simulink model "d2017_10_18_Pendulum"  (R2017b)
settings: Solver=VariableStepAuto  StartTime=0.0  StopTime=30.0  MaxStep=0.01  RelTol=1e-3
settings Model: Creator=ppolcz  LastModifiedBy=ppolcz

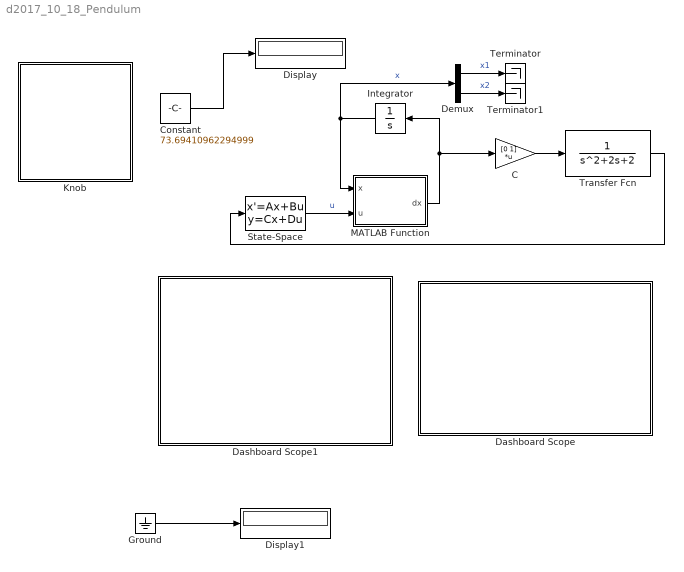
== system d2017_10_18_Pendulum ==
  C : Gain  Gain=[0 1]  Multiplication=Matrix(K*u)
  Constant : Constant  Value=73.69410962294999
  Dashboard Scope : Subsystem  DialogController=hmiCreateDDGDialog  IsWebBlock=on  mask(MWDashboardBlock){webBlockId=452c7a18-fb59-4353-a9f1-2ab489e9cfdd, webBlockType=sdiscope, ShowInitialText=on, HMISrcModelName=d2017_10_18_Pendulum}
      mask prompts: webBlockId "WebBlock Id"; webBlockType "WebBlock Type"; HMISrcModelName "Source Model"
      mask help: SimulinkHMI:dialogs:HMIScopeDialogDesc
      mask Help: helpview([docroot '/mapfiles/simulink.map'], 'hmi_scope')
      mask Display:
      | if strcmp(get_param(bdroot(gcb),'BlockDiagramType'), 'library')
      |     image([(matlabroot) '/toolbox/simulink/hmi/icons/DashboardScope.png']);
      | end
  Dashboard Scope1 : Subsystem  DialogController=hmiCreateDDGDialog  IsWebBlock=on  mask(MWDashboardBlock){webBlockId=a39190fb-05bf-4807-b1f0-982a02af638b, webBlockType=sdiscope, ShowInitialText=on, HMISrcModelName=d2017_10_18_Pendulum}
      mask prompts: webBlockId "WebBlock Id"; webBlockType "WebBlock Type"; HMISrcModelName "Source Model"
      mask help: SimulinkHMI:dialogs:HMIScopeDialogDesc
      mask Help: helpview([docroot '/mapfiles/simulink.map'], 'hmi_scope')
      mask Display:
      | if strcmp(get_param(bdroot(gcb),'BlockDiagramType'), 'library')
      |     image([(matlabroot) '/toolbox/simulink/hmi/icons/DashboardScope.png']);
      | end
  Demux : Demux  Outputs=2
  Display : Display
  Display1 : Display
  Ground : Ground
  Integrator : Integrator  InitialCondition=[0.5;0]
  Knob : Subsystem  DialogController=hmiCreateDDGDialog  IsWebBlock=on  mask(MWDashboardBlock){webBlockId=b0feccf8-7cab-4ec6-92ab-e2df7a33f00f, webBlockType=continuousknob, ShowInLibBrowser=on, ShowInitialText=on, HMISrcModelName=d2017_10_18_Pendulum}
      mask prompts: webBlockId "WebBlock Id"; webBlockType "WebBlock Type"; HMISrcModelName "Source Model"
      mask help: SimulinkHMI:dialogs:ContinuousKnobDialogDesc
      mask Help: helpview([docroot '/mapfiles/simulink.map'], 'hmi_knob')
      mask Display:
      | if strcmp(get_param(bdroot(gcb),'BlockDiagramType'), 'library')
      |     image([(matlabroot) '/toolbox/simulink/hmi/icons/ContinuousKnob.png']);
      | end
  MATLAB Function : MATLAB Function  TreatAsAtomicUnit=on
  State-Space : StateSpace  A=[0 1 ; -1 -0.7]  B=[0 ; 1]  C=[0 1]  D=[0]  InitialCondition=[1;0]
  Terminator : Terminator
  Terminator1 : Terminator
  Transfer Fcn : TransferFcn  Denominator=[1 2 2]
  wires:
  Integrator/1 -> Demux/1, MATLAB Function/1(x)  "x"
  MATLAB Function/1(dx) -> C/1, Integrator/1
  State-Space/1 -> MATLAB Function/2(u)  "u"
  Transfer Fcn/1 -> State-Space/1
  C/1 -> Transfer Fcn/1
  Constant/1 -> Display/1
  Ground/1 -> Display1/1
  Demux/1 -> Terminator/1  "x1"
  Demux/2 -> Terminator1/1  "x2"

== system d2017_10_18_Pendulum/Dashboard Scope ==

== system d2017_10_18_Pendulum/Dashboard Scope1 ==

== system d2017_10_18_Pendulum/Knob ==

== matlab function d2017_10_18_Pendulum/MATLAB Function ==
  data: x input; dx output; u input
function dx = fcn(x,u)

m = 1;
l = 1;
g = 9.8;
b = 0.3;

dx = [
    x(2)
    -g/l*sin(x(1)) - b/m*x(2) + u
    ];

end
